simulink model "AccelSmoothingAndSaturation_4RTMaps"  (R2024a)
settings: Solver=FixedStepDiscrete  StartTime=0.0  StopTime=10.0  FixedStep=0.05  RelTol=1e-3
settings Model: Creator=darkh  LastModifiedBy=darkh
settings OptimizationCC: ZeroExternalMemoryAtStartup=off  ZeroInternalMemoryAtStartup=off
settings RTWCC: Description=Generate an RTMaps component embedding the model  SystemTargetFile=rtmaps.tlc  TemplateMakefile=rtmaps_default_tmf  PostCodeGenCommand=rtmaps_post_code_generation(buildInfo)  RetainRTWFile=on  TargetLang=C++
settings STFCustomTargetCC: TargetLangStandard=C++11 (ISO)  ModelReferenceCompliant=off  ConcurrentExecutionCompliant=on  CombineOutputUpdateFcns=on  CodeInterfacePackaging=C++ class  CPPClassGenCompliant=on  GRTInterface=off  UseToolchainInfoCompliant=off  SystemTargetFile=rtmaps.tlc
settings GRTTargetCC: TargetLangStandard=C++11 (ISO)  ModelReferenceCompliant=off  ParMdlRefBuildCompliant=off  CompOptLevelCompliant=off  MatFileLogging=off  CodeInterfacePackaging=C++ class  UseToolchainInfoCompliant=off

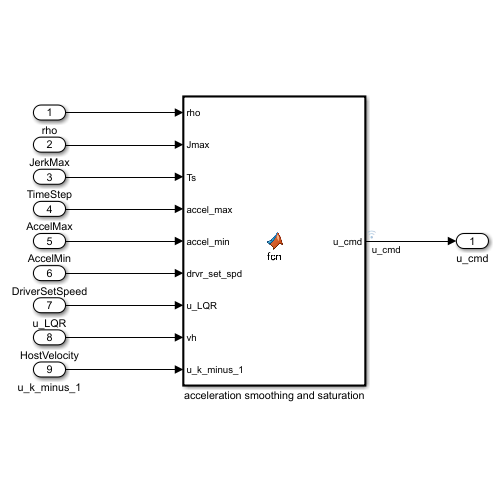
[thumbnail: Simulink's stored preview of the top-level diagram]
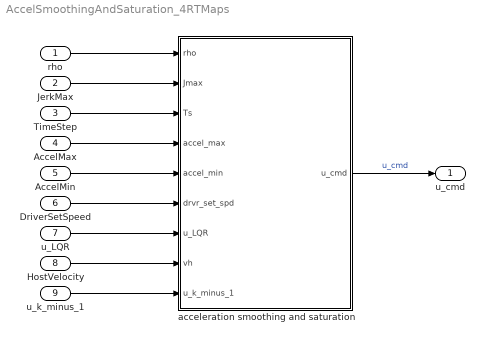
== system AccelSmoothingAndSaturation_4RTMaps ==
  rho : Inport
  JerkMax : Inport  Port=2
  TimeStep : Inport  Port=3
  AccelMax : Inport  Port=4
  AccelMin : Inport  Port=5
  DriverSetSpeed : Inport  Port=6
  u_LQR : Inport  Port=7
  HostVelocity : Inport  Port=8
  u_k_minus_1 : Inport  Port=9
  acceleration smoothing and saturation : MATLAB Function  TreatAsAtomicUnit=on
  u_cmd : Outport
  wires:
  rho/1 -> acceleration smoothing and saturation/1(rho)
  JerkMax/1 -> acceleration smoothing and saturation/2(Jmax)
  TimeStep/1 -> acceleration smoothing and saturation/3(Ts)
  AccelMax/1 -> acceleration smoothing and saturation/4(accel_max)
  AccelMin/1 -> acceleration smoothing and saturation/5(accel_min)
  DriverSetSpeed/1 -> acceleration smoothing and saturation/6(drvr_set_spd)
  u_LQR/1 -> acceleration smoothing and saturation/7(u_LQR)
  HostVelocity/1 -> acceleration smoothing and saturation/8(vh)
  u_k_minus_1/1 -> acceleration smoothing and saturation/9(u_k_minus_1)
  acceleration smoothing and saturation/1(u_cmd) -> u_cmd/1  "u_cmd"

== matlab function AccelSmoothingAndSaturation_4RTMaps/acceleration smoothing and saturation ==
  data: rho input; Jmax input; Ts input; accel_max input; accel_min input; drvr_set_spd input; u_cmd output; u_LQR input; vh input; u_k_minus_1 input
function u_cmd = fcn(rho, Jmax, Ts, accel_max, accel_min, drvr_set_spd, u_LQR, vh, u_k_minus_1)

u_tilde = (u_LQR + rho*u_k_minus_1)/(1 + rho);

u_cmd = min(max(u_tilde, u_k_minus_1 - Jmax*Ts), u_k_minus_1 + Jmax*Ts); 
u_cmd = min(max(u_cmd, accel_min), accel_max); 

if (vh <= 0.001 && u_cmd < 0.0) 
    u_cmd = 0.0;
elseif (vh >= drvr_set_spd && u_cmd > 0.0)
    alpha = exp(-Ts/0.5);
    u_cmd = alpha*u_k_minus_1 + (1-alpha)*0.0;
end
